simulink model "sway_elastic_sim"  (R2020a)
settings: Solver=VariableStepAuto  StartTime=0.0  StopTime=10  RelTol=1e-3
values from neighbouring files (symbols this model uses):
  Ag = 1    [sway_elastic.m]
  g = 9.8    [sway_elastic.m]
  ig1_init = 0    [sway_elastic.m]
  ig3_init = 0    [sway_elastic.m]
  ig4_init = 0    [sway_elastic.m]
  Jz = 2853*10^3    (= 2853000)    [sway_elastic.m]
  K = lqr(A,B,Q,Rr)    [sway_elastic.m]
  l = 8    [Shape_Function.m]    (also in sway_elastic.m)
  m = 60000    [sway_elastic.m]
  mu0 = 1.25*10^-6    (= 1.25e-06)    [sway_elastic.m]
  Ng = 500    [sway_elastic.m]
  P1 = 100    [sway_elastic.m]
  P2 = 100    [sway_elastic.m]
  P3 = 100    [sway_elastic.m]
  P4 = 100    [sway_elastic.m]
  P5 = 100    [sway_elastic.m]
  P6 = 100    [sway_elastic.m]
  phi = 0    [sway_elastic.m]
  PHI12 = eval(PHI)    [sway_elastic.m]
  PHI20 = eval(PHI)    [sway_elastic.m]
  PHI4 = eval(PHI)    [sway_elastic.m]
  PHIc = eval(int21)    [sway_elastic.m]
  PHIf = eval(int11)    [sway_elastic.m]
  PHIr = eval(int31)    [sway_elastic.m]
  psi_init = 0    [sway_elastic.m]
  ql_init = 0    [sway_elastic.m]
  R = diag([weight_Vg1 weight_Vg2 weight_Vg3 weight_Vg4 weight_Vg5 weight_Vg6])    [sway_elastic.m]
  Ra = 0    [sway_elastic.m]
  vql_init = 0    [sway_elastic.m]
  Vref = [ Vg1; Vg2; Vg3; Vg4; Vg5; Vg6]    [sway_elastic.m]
  vx = 430/3.6    (= 119.444444444)    [sway_elastic.m]
  vy_init = 0    [sway_elastic.m]
  w = eval(omega_1)    [sway_elastic.m]
  wpsi = 0    [sway_elastic.m]
  wpsi_init = 0    [sway_elastic.m]
  x_ref = [y_ref; vy_ref; psi_ref; wpsi_ref; ig_ref; ig_ref; ig_ref; ig_ref; ig_ref; ig_ref; ql_ref; vql_ref]    [sway_elastic.m]
  xB = 8    [sway_elastic.m]
  y_init = 0.01    [sway_elastic.m]
  yB = 2    [sway_elastic.m]
  ymax = 0.02    [sway_elastic.m]
settings Model: Creator=Federico  LastModifiedBy=Federico

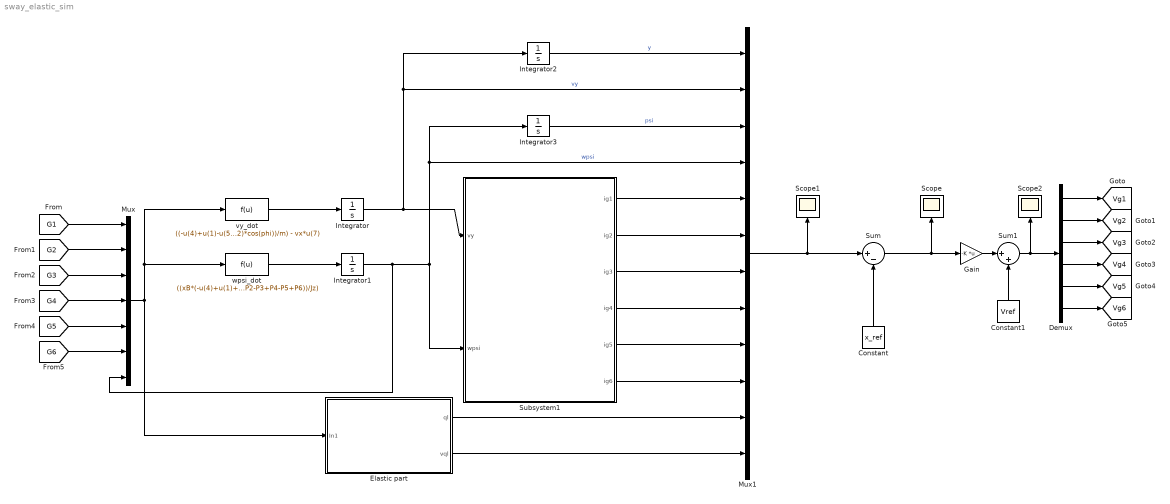
== system sway_elastic_sim ==
  Constant : Constant  Value=x_ref
  Constant1 : Constant  Value=Vref
  Demux : Demux  Outputs=6
  Elastic part : Subsystem
  Gain : Gain  Gain=-K  Multiplication=Matrix(K*u)
  Integrator : Integrator  InitialCondition=vy_init
  Integrator1 : Integrator  InitialCondition=wpsi_init
  Integrator2 : Integrator  InitialCondition=y_init
  Integrator3 : Integrator  InitialCondition=psi_init
  Mux : Mux  Inputs=7
  Mux1 : Mux  Inputs=12
  Scope : Scope
  Scope1 : Scope
  Scope2 : Scope
  Subsystem1 : Subsystem
  Sum : Sum  Inputs=|+-
  Sum1 : Sum  Inputs=|++
  vy_dot : Fcn  Expr=((-u(4)+u(1)-u(5)+u(2)-u(6)+u(3)+m*g*sin(phi)-m*Ra*(wpsi^2)*cos(phi))/m) - vx*u(7)
  wpsi_dot : Fcn  Expr=((xB*(-u(4)+u(1)+u(6)-u(3))+yB*(-P1+P2-P3+P4-P5+P6))/Jz)
  tag scope: Vg1=global, Vg2=global, Vg3=global, Vg4=global, Vg5=global, Vg6=global
  wires:
  vy_dot/1 -> Integrator/1
  wpsi_dot/1 -> Integrator1/1
  Integrator/1 -> Integrator2/1, Mux1/2, Subsystem1/1(vy)  "vy"
  Integrator1/1 -> Mux/7, Integrator3/1, Mux1/4, Subsystem1/2(wpsi)  "wpsi"
  Mux/1 -> wpsi_dot/1, vy_dot/1, Elastic part/1(In1)
  [G1] -> Mux/1
  [G2] -> Mux/2
  [G3] -> Mux/3
  [G4] -> Mux/4
  [G5] -> Mux/5
  [G6] -> Mux/6
  Integrator2/1 -> Mux1/1  "y"
  Integrator3/1 -> Mux1/3  "psi"
  Subsystem1/1(ig1) -> Mux1/5
  Subsystem1/2(ig2) -> Mux1/6
  Subsystem1/3(ig3) -> Mux1/7
  Subsystem1/4(ig4) -> Mux1/8
  Subsystem1/5(ig5) -> Mux1/9
  Subsystem1/6(ig6) -> Mux1/10
  Demux/1 -> [Vg1]
  Demux/2 -> [Vg2]
  Demux/4 -> [Vg4]
  Demux/3 -> [Vg3]
  Demux/5 -> [Vg5]
  Demux/6 -> [Vg6]
  Elastic part/1(ql) -> Mux1/11
  Elastic part/2(vql) -> Mux1/12
  Mux1/1 -> Sum/1, Scope1/1
  Sum/1 -> Gain/1, Scope/1
  Gain/1 -> Sum1/1
  Sum1/1 -> Scope2/1, Demux/1
  Constant/1 -> Sum/2
  Constant1/1 -> Sum1/2

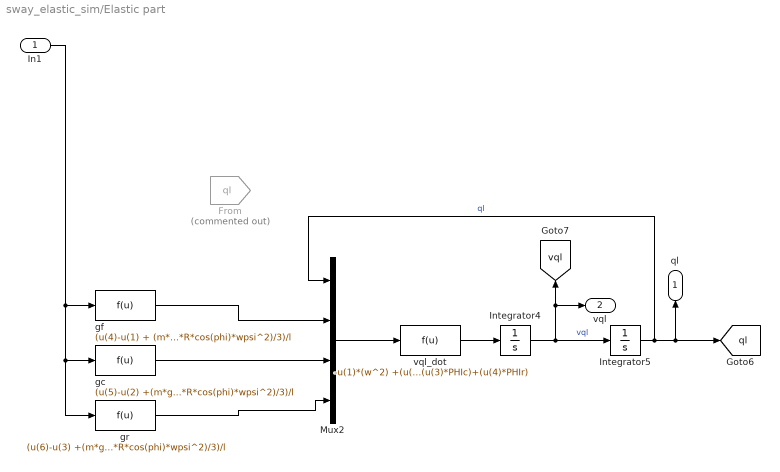
== system sway_elastic_sim/Elastic part ==
  In1 : Inport
  From : From  Commented=on  GotoTag=ql  TagVisibility=global
  Integrator4 : Integrator  InitialCondition=vql_init
  Integrator5 : Integrator  InitialCondition=ql_init
  Mux2 : Mux
  gc : Fcn  Expr=(u(5)-u(2) +(m*g*sin(phi)-m*R*cos(phi)*wpsi^2)/3)/l
  gf : Fcn  Expr=(u(4)-u(1) + (m*g*sin(phi)-m*R*cos(phi)*wpsi^2)/3)/l
  gr : Fcn  Expr=(u(6)-u(3) +(m*g*sin(phi)-m*R*cos(phi)*wpsi^2)/3)/l
  vql_dot : Fcn  Expr=-u(1)*(w^2) +(u(2)*PHIf)+(u(3)*PHIc)+(u(4)*PHIr)
  ql : Outport
  vql : Outport  Port=2
  tag scope: ql=global, vql=global
  wires:
  Integrator5/1 -> Mux2/1, [ql], ql/1  "ql"
  Integrator4/1 -> Integrator5/1, vql/1, [vql]  "vql"
  gr/1 -> Mux2/4
  In1/1 -> gr/1, gc/1, gf/1
  Mux2/1 -> vql_dot/1
  gf/1 -> Mux2/2
  gc/1 -> Mux2/3
  vql_dot/1 -> Integrator4/1

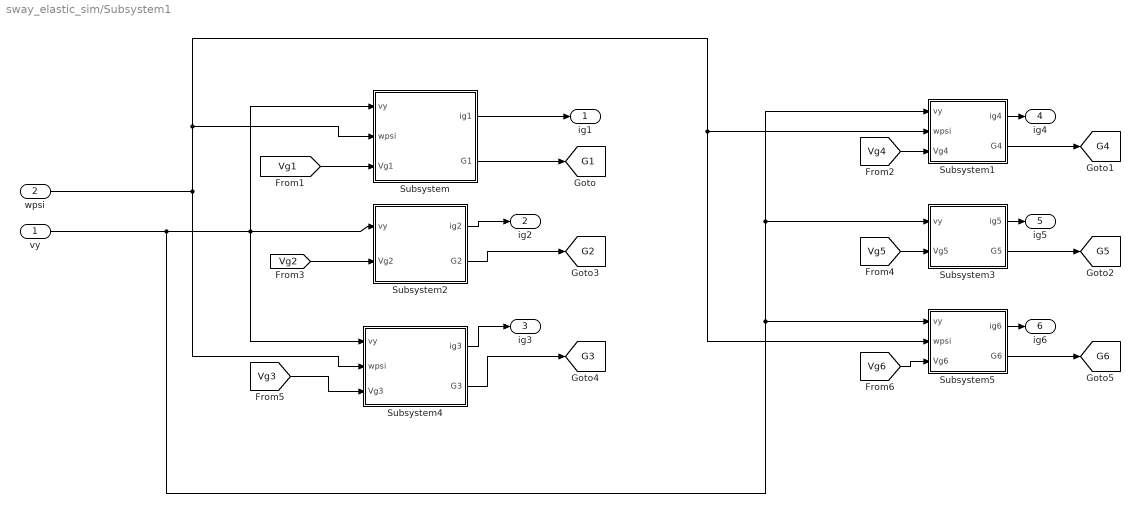
== system sway_elastic_sim/Subsystem1 ==
  vy : Inport
  wpsi : Inport  Port=2
  Subsystem : Subsystem
  Subsystem1 : Subsystem
  Subsystem2 : Subsystem
  Subsystem3 : Subsystem
  Subsystem4 : Subsystem
  Subsystem5 : Subsystem
  ig1 : Outport
  ig2 : Outport  Port=2
  ig3 : Outport  Port=3
  ig4 : Outport  Port=4
  ig5 : Outport  Port=5
  ig6 : Outport  Port=6
  tag scope: G1=global, G2=global, G3=global, G4=global, G5=global, G6=global
  wires:
  Subsystem/2(G1) -> [G1]
  [Vg3] -> Subsystem4/3(Vg3)
  [Vg1] -> Subsystem/3(Vg1)
  Subsystem4/1(ig3) -> ig3/1
  Subsystem/1(ig1) -> ig1/1
  Subsystem2/1(ig2) -> ig2/1
  Subsystem2/2(G2) -> [G2]
  [Vg2] -> Subsystem2/2(Vg2)
  Subsystem4/2(G3) -> [G3]
  Subsystem5/2(G6) -> [G6]
  [Vg5] -> Subsystem3/2(Vg5)
  wpsi/1 -> Subsystem5/2(wpsi), Subsystem1/2(wpsi), Subsystem/2(wpsi), Subsystem4/2(wpsi)
  Subsystem3/2(G5) -> [G5]
  Subsystem3/1(ig5) -> ig5/1
  Subsystem1/1(ig4) -> ig4/1
  Subsystem5/1(ig6) -> ig6/1
  [Vg4] -> Subsystem1/3(Vg4)
  [Vg6] -> Subsystem5/3(Vg6)
  Subsystem1/2(G4) -> [G4]
  vy/1 -> Subsystem/1(vy), Subsystem2/1(vy), Subsystem4/1(vy), Subsystem1/1(vy), Subsystem3/1(vy), Subsystem5/1(vy)

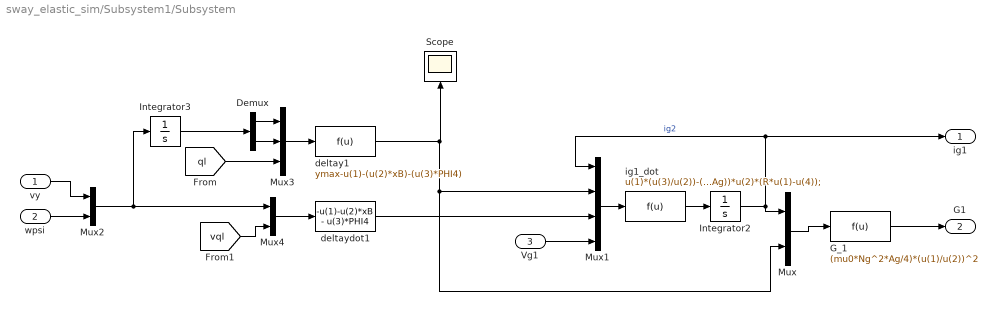
== system sway_elastic_sim/Subsystem1/Subsystem ==
  vy : Inport
  wpsi : Inport  Port=2
  Vg1 : Inport  Port=3
  Demux : Demux  Outputs=2
  G_1 : Fcn  Expr=(mu0*Ng^2*Ag/4)*(u(1)/u(2))^2
  Integrator2 : Integrator  InitialCondition=ig1_init
  Integrator3 : Integrator  InitialCondition=[y_init; psi_init]
  Mux : Mux  Inputs=2
  Mux1 : Mux
  Mux2 : Mux  Inputs=2
  Mux3 : Mux  Inputs=3
  Mux4 : Mux  Inputs=2
  Scope : Scope
  deltay1 : Fcn  Expr=ymax-u(1)-(u(2)*xB)-(u(3)*PHI4)
  deltaydot1 : Fcn  Expr=-u(1)-u(2)*xB - u(3)*PHI4
  ig1_dot : Fcn  Expr=u(1)*(u(3)/u(2))-(2/(mu0*(Ng^2)*Ag))*u(2)*(R*u(1)-u(4));
  ig1 : Outport
  G1 : Outport  Port=2
  wires:
  ig1_dot/1 -> Integrator2/1
  G_1/1 -> G1/1
  deltaydot1/1 -> Mux1/3
  vy/1 -> Mux2/1
  Mux2/1 -> Mux4/1, Integrator3/1
  Vg1/1 -> Mux1/4
  Mux/1 -> G_1/1
  Integrator2/1 -> Mux/1, ig1/1, Mux1/1  "ig2"
  wpsi/1 -> Mux2/2
  Mux1/1 -> ig1_dot/1
  deltay1/1 -> Mux1/2, Mux/2, Scope/1
  Mux3/1 -> deltay1/1
  Mux4/1 -> deltaydot1/1
  [ql] -> Mux3/3
  [vql] -> Mux4/2
  Integrator3/1 -> Demux/1
  Demux/1 -> Mux3/1
  Demux/2 -> Mux3/2

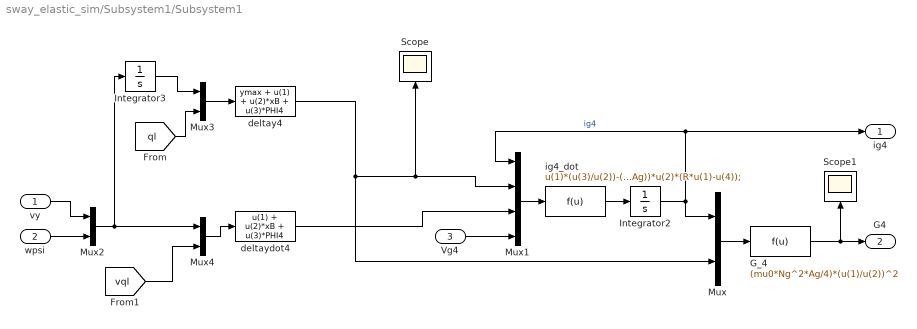
== system sway_elastic_sim/Subsystem1/Subsystem1 ==
  vy : Inport
  wpsi : Inport  Port=2
  Vg4 : Inport  Port=3
  G_4 : Fcn  Expr=(mu0*Ng^2*Ag/4)*(u(1)/u(2))^2
  Integrator2 : Integrator  InitialCondition=ig1_init
  Integrator3 : Integrator  InitialCondition=[y_init; psi_init]
  Mux{,2..4} (4 alike) : Mux  Inputs=2
  Mux1 : Mux
  Scope : Scope
  Scope1 : Scope
  deltay4 : Fcn  Expr=ymax + u(1) + u(2)*xB + u(3)*PHI4
  deltaydot4 : Fcn  Expr=u(1) + u(2)*xB + u(3)*PHI4
  ig4_dot : Fcn  Expr=u(1)*(u(3)/u(2))-(2/(mu0*(Ng^2)*Ag))*u(2)*(R*u(1)-u(4));
  ig4 : Outport
  G4 : Outport  Port=2
  wires:
  deltay4/1 -> Mux/2, Mux1/2, Scope/1
  Mux1/1 -> ig4_dot/1
  wpsi/1 -> Mux2/2
  Integrator2/1 -> Mux1/1, ig4/1, Mux/1  "ig4"
  Mux/1 -> G_4/1
  Vg4/1 -> Mux1/4
  Mux2/1 -> Mux4/1, Integrator3/1
  vy/1 -> Mux2/1
  deltaydot4/1 -> Mux1/3
  G_4/1 -> Scope1/1, G4/1
  ig4_dot/1 -> Integrator2/1
  Integrator3/1 -> Mux3/1
  Mux3/1 -> deltay4/1
  [ql] -> Mux3/2
  Mux4/1 -> deltaydot4/1
  [vql] -> Mux4/2

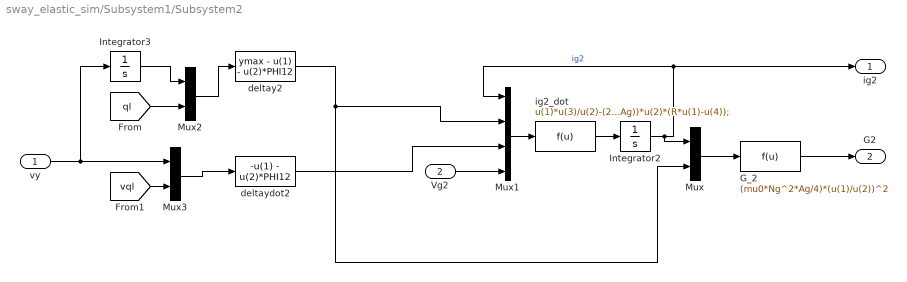
== system sway_elastic_sim/Subsystem1/Subsystem2 ==
  vy : Inport
  Vg2 : Inport  Port=2
  G_2 : Fcn  Expr=(mu0*Ng^2*Ag/4)*(u(1)/u(2))^2
  Integrator2 : Integrator  InitialCondition=ig4_init
  Integrator3 : Integrator  InitialCondition=y_init
  Mux : Mux  Inputs=2
  Mux1 : Mux
  Mux2 : Mux  Inputs=2
  Mux3 : Mux  Inputs=2
  deltay2 : Fcn  Expr=ymax - u(1) - u(2)*PHI12
  deltaydot2 : Fcn  Expr=-u(1) - u(2)*PHI12
  ig2_dot : Fcn  Expr=u(1)*u(3)/u(2)-(2/(mu0*(Ng^2)*Ag))*u(2)*(R*u(1)-u(4));
  ig2 : Outport
  G2 : Outport  Port=2
  wires:
  deltay2/1 -> Mux/2, Mux1/2
  Mux1/1 -> ig2_dot/1
  Integrator2/1 -> Mux/1, Mux1/1, ig2/1  "ig2"
  Mux/1 -> G_2/1
  Vg2/1 -> Mux1/4
  deltaydot2/1 -> Mux1/3
  G_2/1 -> G2/1
  ig2_dot/1 -> Integrator2/1
  vy/1 -> Mux3/1, Integrator3/1
  Mux2/1 -> deltay2/1
  Integrator3/1 -> Mux2/1
  [ql] -> Mux2/2
  Mux3/1 -> deltaydot2/1
  [vql] -> Mux3/2

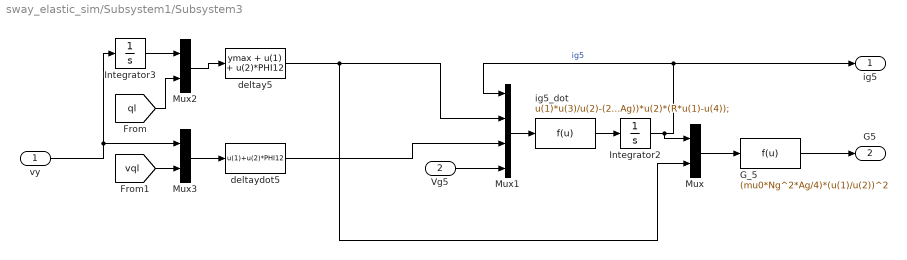
== system sway_elastic_sim/Subsystem1/Subsystem3 ==
  vy : Inport
  Vg5 : Inport  Port=2
  G_5 : Fcn  Expr=(mu0*Ng^2*Ag/4)*(u(1)/u(2))^2
  Integrator2 : Integrator  InitialCondition=ig4_init
  Integrator3 : Integrator  InitialCondition=y_init
  Mux : Mux  Inputs=2
  Mux1 : Mux
  Mux2 : Mux  Inputs=2
  Mux3 : Mux  Inputs=2
  deltay5 : Fcn  Expr=ymax + u(1) + u(2)*PHI12
  deltaydot5 : Fcn  Expr=u(1)+u(2)*PHI12
  ig5_dot : Fcn  Expr=u(1)*u(3)/u(2)-(2/(mu0*(Ng^2)*Ag))*u(2)*(R*u(1)-u(4));
  ig5 : Outport
  G5 : Outport  Port=2
  wires:
  vy/1 -> Mux3/1, Integrator3/1
  ig5_dot/1 -> Integrator2/1
  G_5/1 -> G5/1
  deltaydot5/1 -> Mux1/3
  Vg5/1 -> Mux1/4
  Mux/1 -> G_5/1
  Integrator2/1 -> ig5/1, Mux1/1, Mux/1  "ig5"
  Mux1/1 -> ig5_dot/1
  deltay5/1 -> Mux/2, Mux1/2
  Integrator3/1 -> Mux2/1
  Mux2/1 -> deltay5/1
  [ql] -> Mux2/2
  Mux3/1 -> deltaydot5/1
  [vql] -> Mux3/2

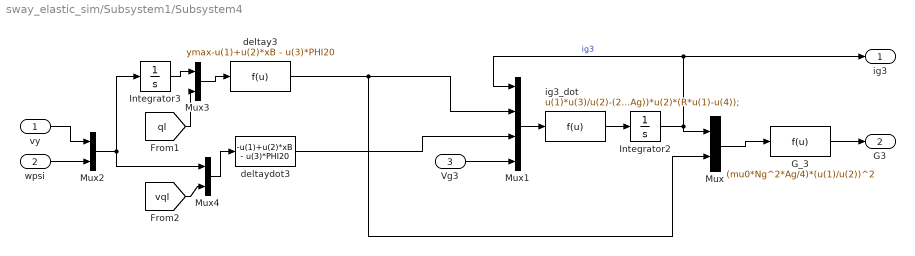
== system sway_elastic_sim/Subsystem1/Subsystem4 ==
  vy : Inport
  wpsi : Inport  Port=2
  Vg3 : Inport  Port=3
  G_3 : Fcn  Expr=(mu0*Ng^2*Ag/4)*(u(1)/u(2))^2
  Integrator2 : Integrator  InitialCondition=ig3_init
  Integrator3 : Integrator  InitialCondition=[y_init; psi_init]
  Mux{,2..4} (4 alike) : Mux  Inputs=2
  Mux1 : Mux
  deltay3 : Fcn  Expr=ymax-u(1)+u(2)*xB - u(3)*PHI20
  deltaydot3 : Fcn  Expr=-u(1)+u(2)*xB - u(3)*PHI20
  ig3_dot : Fcn  Expr=u(1)*u(3)/u(2)-(2/(mu0*(Ng^2)*Ag))*u(2)*(R*u(1)-u(4));
  ig3 : Outport
  G3 : Outport  Port=2
  wires:
  ig3_dot/1 -> Integrator2/1
  G_3/1 -> G3/1
  deltaydot3/1 -> Mux1/3
  vy/1 -> Mux2/1
  Mux2/1 -> Integrator3/1, Mux4/1
  Vg3/1 -> Mux1/4
  Mux/1 -> G_3/1
  Integrator2/1 -> ig3/1, Mux1/1, Mux/1  "ig3"
  wpsi/1 -> Mux2/2
  deltay3/1 -> Mux/2, Mux1/2
  Mux1/1 -> ig3_dot/1
  Mux3/1 -> deltay3/1
  Integrator3/1 -> Mux3/1
  [ql] -> Mux3/2
  [vql] -> Mux4/2
  Mux4/1 -> deltaydot3/1

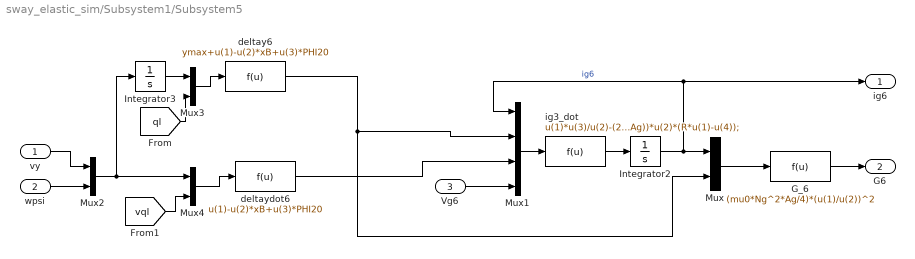
== system sway_elastic_sim/Subsystem1/Subsystem5 ==
  vy : Inport
  wpsi : Inport  Port=2
  Vg6 : Inport  Port=3
  G_6 : Fcn  Expr=(mu0*Ng^2*Ag/4)*(u(1)/u(2))^2
  Integrator2 : Integrator  InitialCondition=ig3_init
  Integrator3 : Integrator  InitialCondition=[y_init; psi_init]
  Mux{,2..4} (4 alike) : Mux  Inputs=2
  Mux1 : Mux
  deltay6 : Fcn  Expr=ymax+u(1)-u(2)*xB+u(3)*PHI20
  deltaydot6 : Fcn  Expr=u(1)-u(2)*xB+u(3)*PHI20
  ig3_dot : Fcn  Expr=u(1)*u(3)/u(2)-(2/(mu0*(Ng^2)*Ag))*u(2)*(R*u(1)-u(4));
  ig6 : Outport
  G6 : Outport  Port=2
  wires:
  deltay6/1 -> Mux/2, Mux1/2
  Integrator3/1 -> Mux3/1
  Mux1/1 -> ig3_dot/1
  wpsi/1 -> Mux2/2
  Integrator2/1 -> Mux/1, Mux1/1, ig6/1  "ig6"
  Mux/1 -> G_6/1
  Vg6/1 -> Mux1/4
  Mux2/1 -> Integrator3/1, Mux4/1
  vy/1 -> Mux2/1
  deltaydot6/1 -> Mux1/3
  G_6/1 -> G6/1
  ig3_dot/1 -> Integrator2/1
  Mux3/1 -> deltay6/1
  [ql] -> Mux3/2
  Mux4/1 -> deltaydot6/1
  [vql] -> Mux4/2
